simulink model "atrias_boom_nmSt_kinSw_v2"  (R2015a)
settings: Solver=ode23t  StartTime=0.0  StopTime=t_end  FixedStep=0.001  MaxStep=1e-3  RelTol=1e-3
InitFcn:
  | addpath('../common/')
  | colors
StartFcn:
  | tic
StopFcn:
  | %stopscript
values from neighbouring files (symbols this model uses):
  dt_a_dTrunk_boom = 5    [main_1_nmSt_kinSw.m]    (also in main_2_nmSt_kinSw_v2.m; main_3_nmSt_kinSw_v3.m; main_4_nmSt_kinSw_v4.m)
  dt_fade_boomCtrl = 2    [main_1_nmSt_kinSw.m]    (also in main_2_nmSt_kinSw_v2.m; main_3_nmSt_kinSw_v3.m; main_4_nmSt_kinSw_v4.m)
  initial_boom_yaw = 15*pi/180    (= 0.261799387799)    [main_2_nmSt_kinSw_v2.m]    (also in main_3_nmSt_kinSw_v3.m; main_4_nmSt_kinSw_v4.m)
  kd_boom_roll_Ctrl = 0    [main_1_nmSt_kinSw - Copy.m]    (also in main_1_nmSt_kinSw.m; main_2_nmSt_kinSw_v2.m; main_3_nmSt_kinSw_v3.m; main_4_nmSt_kinSw_v4.m)
  kd_boom_yaw_Ctrl = 0.1*kp_boom_yaw_Ctrl    (= 100000000)    [main_1_nmSt_kinSw - Copy.m]    (also in main_1_nmSt_kinSw.m = 1000000000; main_2_nmSt_kinSw_v2.m = 10000000; main_3_nmSt_kinSw_v3.m = 10000000; main_4_nmSt_kinSw_v4.m = 10000000)
  kd_motor = 0.90*2*sqrt(3.75*kp_motor)    [main_1_nmSt_kinSw - Copy.m]
  kinSw_alpha_start = 100*pi/180    (= 1.74532925199)    [main_1_nmSt_kinSw - Copy.m]    (also in main_1_nmSt_kinSw.m = 1.91986217719; main_2_nmSt_kinSw_v2.m = 1.83259571459; main_3_nmSt_kinSw_v3.m = 1.83259571459; main_4_nmSt_kinSw_v4.m = 1.83259571459)
  kinSw_alpha_tgt = 80*pi/180    (= 1.3962634016)    [main_1_nmSt_kinSw - Copy.m]    (also in main_1_nmSt_kinSw.m = 1.2217304764; main_2_nmSt_kinSw_v2.m = 1.2217304764; main_3_nmSt_kinSw_v3.m = 1.2217304764; main_4_nmSt_kinSw_v4.m = 1.2217304764)
  kinSw_t_start = 1.5    [main_1_nmSt_kinSw - Copy.m]    (also in main_1_nmSt_kinSw.m; main_2_nmSt_kinSw_v2.m = 0.5; main_3_nmSt_kinSw_v3.m = 0.5; main_4_nmSt_kinSw_v4.m = 0.5)
  kp_boom_roll_Ctrl = 0    [main_1_nmSt_kinSw - Copy.m]    (also in main_1_nmSt_kinSw.m; main_2_nmSt_kinSw_v2.m; main_3_nmSt_kinSw_v3.m; main_4_nmSt_kinSw_v4.m)
  kp_boom_yaw_Ctrl = 1e9    (= 1000000000)    [main_1_nmSt_kinSw - Copy.m]    (also in main_1_nmSt_kinSw.m = 10000000000; main_2_nmSt_kinSw_v2.m = 100000000; main_3_nmSt_kinSw_v3.m = 100000000; main_4_nmSt_kinSw_v4.m = 100000000)
  kp_motor = 3000    [main_1_nmSt_kinSw - Copy.m]
  max_back_bar_angle = 262.4*pi/180    (= 4.57974395723)    [main_1_nmSt_kinSw - Copy.m]
  max_front_bar_angle = 194.8*pi/180    (= 3.39990138288)    [main_1_nmSt_kinSw - Copy.m]
  min_back_bar_angle = 165.0*pi/180    (= 2.87979326579)    [main_1_nmSt_kinSw - Copy.m]
  min_front_bar_angle = 98.0*pi/180    (= 1.71042266695)    [main_1_nmSt_kinSw - Copy.m]
  poser_LLegAlp = (initial_l_leg_angle -pi/2)*180/pi    (= 105)    [main_2_nmSt_kinSw_v2.m]    (also in main_3_nmSt_kinSw_v3.m; main_4_nmSt_kinSw_v4.m)
  poser_LLegLen = initial_l_leg_length    (= 0.88)    [main_2_nmSt_kinSw_v2.m]    (also in main_3_nmSt_kinSw_v3.m; main_4_nmSt_kinSw_v4.m)
  poser_RLegAlp = (initial_r_leg_angle -pi/2)*180/pi    (= 75)    [main_2_nmSt_kinSw_v2.m]    (also in main_3_nmSt_kinSw_v3.m; main_4_nmSt_kinSw_v4.m)
  poser_RLegLen = initial_r_leg_length    (= 0.9)    [main_2_nmSt_kinSw_v2.m]    (also in main_3_nmSt_kinSw_v3.m; main_4_nmSt_kinSw_v4.m)
  tEnd_boomCtrl = t_end    (= 20)    [main_1_nmSt_kinSw - Copy.m]    (also in main_1_nmSt_kinSw.m = 3; main_2_nmSt_kinSw_v2.m = 7.5; main_3_nmSt_kinSw_v3.m = 7.5; main_4_nmSt_kinSw_v4.m = 7.5)
  tStart_boomCtrl = 1    [main_1_nmSt_kinSw - Copy.m]    (also in main_1_nmSt_kinSw.m = 0; main_2_nmSt_kinSw_v2.m = 0.5; main_3_nmSt_kinSw_v3.m = 0.5; main_4_nmSt_kinSw_v4.m = 0.5)
  tune_kinSw_alpha_start = kinSw_alpha_start*180/pi    (= 105)    [main_2_nmSt_kinSw_v2.m]    (also in main_3_nmSt_kinSw_v3.m; main_4_nmSt_kinSw_v4.m)
  tune_kinSw_alpha_tgt = kinSw_alpha_tgt*180/pi    (= 70)    [main_2_nmSt_kinSw_v2.m]    (also in main_3_nmSt_kinSw_v3.m; main_4_nmSt_kinSw_v4.m)
  tune_kinSw_len_min = kinSw_lclr    (= 0.7)    [main_2_nmSt_kinSw_v2.m]    (also in main_3_nmSt_kinSw_v3.m = 0.6)
  tune_kinSw_len_tgt = kinSw_len_tgt    (= 0.9)    [main_2_nmSt_kinSw_v2.m]    (also in main_3_nmSt_kinSw_v3.m)
  tune_M1_G = St_FGain_VAS*FmaxVAS    [main_2_nmSt_kinSw_v2.m]    (also in main_3_nmSt_kinSw_v3.m; main_4_nmSt_kinSw_v4.m)
  tune_M3_0 = CtrlPar_theta0*180/pi    [main_2_nmSt_kinSw_v2.m]    (also in main_3_nmSt_kinSw_v3.m; main_4_nmSt_kinSw_v4.m)
  tune_M3_D = St_GainDTh_HFL    [main_2_nmSt_kinSw_v2.m]    (also in main_3_nmSt_kinSw_v3.m; main_4_nmSt_kinSw_v4.m)
  tune_M3_P = St_GainTh_HFL    [main_2_nmSt_kinSw_v2.m]    (also in main_3_nmSt_kinSw_v3.m; main_4_nmSt_kinSw_v4.m)
  v_dTrunk_boom = 1.3    [main_1_nmSt_kinSw.m]    (also in main_2_nmSt_kinSw_v2.m; main_3_nmSt_kinSw_v3.m; main_4_nmSt_kinSw_v4.m)
undefined symbols (not defined in the file or in its folder): A1_notch_f1, A2_notch_f1, A_lpf_dtau, A_lpf_velocity, ankle_stiffness, B1_lpf_dtau, B1_lpf_velocity, B1_notch_f1, B2_lpf_dtau, B2_lpf_velocity, B2_notch_f1, b_hmotor, b_leg_spring, b_rotor, base_color_d, boom_color_d, boom_mount_to_center_diagonal, breakaway_friction, c_jointstop, contactThr, coulomb_friction, d_com, delta_phi_max, delta_phi_max_buffer, delta_phi_max_dropoff, delta_phi_min, fblink_color_d, floor_color_d, FmaxBFSH, FmaxGLU, FmaxHAM, FmaxHFL, FmaxRF, FmaxVAS, foot_color_d, FPCtrlPar, friction_linear_zone, g, gain_nodes_sea_torque, HIP_MTR_MAX_CONT_TORQUE, HIP_MTR_MAX_TORQUE, hshaft_color_d, initial_boom_pitch, initial_boom_roll, initial_hip_roll, initial_winch_angle, j_motor, k_gn, k_gt, k_leg_spring, K_notch_f1, k_phi, k_sea, Kb_leg, kd_lateral, kd_shin_max, kd_shin_min, kd_splay_max, kd_splay_min, kd_thigh_max ... (+187)
libraries: sm_lib x210, nesl_utility x140, simulink x65, simulink_extras x31, fl_lib x16, mblibv1 x2, commnoisgen2 x1
(part 3 of 16)

== system atrias_boom_nmSt_kinSw_v2/Mechanical System Layer/Left Foot ==
  Ankle : sm_lib/Joints/Revolute Joint  SenseConstraintForce=off  SenseConstraintForceX=off  SenseConstraintForceY=off  SenseConstraintForceZ=off  SenseConstraintTorque=off  SenseConstraintTorqueX=off  SenseConstraintTorqueY=off  SenseConstraintTorqueZ=off  SenseTotalForce=off  SenseTotalForceX=off  SenseTotalForceY=off  SenseTotalForceZ=off  SenseTotalTorque=off  SenseTotalTorqueX=off  SenseTotalTorqueY=off  SenseTotalTorqueZ=off  CompositeWrenchDir=FollowerOnBase  CompositeWrenchFrame=BaseFrame  EquilibriumPosition=ankle_equilibrium  EquilibriumPositionUnits=rad  SpringStiffness=ankle_stiffness  SpringStiffnessUnits=N*m/rad  DampingCoefficient=0.1*ankle_stiffness  DampingCoefficientUnits=N*m/(rad/s)  TorqueActuationMode=NoTorque  MotionActuationMode=ComputedMotion  SensePosition=off  SenseVelocity=off  SenseAcceleration=off  SenseTorqueForce=off  PositionTargetSpecify=on  PositionTargetPriority=Low  PositionTargetValue=ankle_initial_l  PositionTargetValueUnits=rad  VelocityTargetSpecify=off  VelocityTargetPriority=High  VelocityTargetValue=6000  VelocityTargetValueUnits=deg/s  BlockFunction=simmechanics.library.joints.revolute_joint
  CS1 to Back Point : sm_lib/Frames and Transforms/Rigid Transform  TranslationMethod=Cartesian  TranslationLengthUnit=m  TranslationStandardAxis=+Z  TranslationStandardOffset=0  TranslationCartesianOffset=d_foot_point_back  TranslationROffset=0  TranslationROffsetUnits=m  TranslationZOffset=0  TranslationZOffsetUnits=m  TranslationThetaOffset=0  TranslationThetaOffsetUnits=deg  RotationMethod=None  RotationAngleUnits=deg  RotationStandardAxis=+Z  RotationAngle=0  RotationArbitraryAxis=[0 0 1]  FollAlignAxisA=+X  BaseAlignAxisA=+Y  FollAlignAxisB=+Y  BaseAlignAxisB=+Z  RotationMatrix=[1 0 0; 0 1 0; 0 0 1]  BlockFunction=simmechanics.library.frames_transforms.rigid_transform
  CS1 to Front Point : sm_lib/Frames and Transforms/Rigid Transform  TranslationMethod=Cartesian  TranslationLengthUnit=m  TranslationStandardAxis=+Z  TranslationStandardOffset=0  TranslationCartesianOffset=d_foot_point_front  TranslationROffset=0  TranslationROffsetUnits=m  TranslationZOffset=0  TranslationZOffsetUnits=m  TranslationThetaOffset=0  TranslationThetaOffsetUnits=deg  RotationMethod=None  RotationAngleUnits=deg  RotationStandardAxis=+Z  RotationAngle=0  RotationArbitraryAxis=[0 0 1]  FollAlignAxisA=+X  BaseAlignAxisA=+Y  FollAlignAxisB=+Y  BaseAlignAxisB=+Z  RotationMatrix=[1 0 0; 0 1 0; 0 0 1]  BlockFunction=simmechanics.library.frames_transforms.rigid_transform
  Solid : sm_lib/Body Elements/Solid  InertiaType=Custom  Mass=m_foot  MassUnits=kg  CenterOfMass=com_foot  CenterOfMassUnits=m  MomentsOfInertia=i_foot_moments  MomentsOfInertiaUnits=kg*m^2  ProductsOfInertia=i_foot_products  ProductsOfInertiaUnits=kg*m^2  DensityBased=on  Density=1000  DensityUnits=kg/(m^3)  GraphicType=FromGeometry  MarkerShape=Sphere  MarkerSize=10  MarkerSizeUnits=m  GraphicVisPropType=AdvancedVisualProperties  GraphicDiffuseColor=foot_color_d  GraphicSpecularColor=[0.5 0.5 0.5 1.0]  GraphicAmbientColor=[foot_color_d*0.5 1.0]  GraphicEmissiveColor=[0.0 0.0 0.0 1.0]  GraphicShininess=128  GraphicOpacity=1.0  GeometryShape=FromFile  RectangleSize=[1 1]  RectangleSizeUnits=m  BrickDimensions=[0.1 l_seg 0.1]  BrickDimensionUnits=m  CylinderRadius=l_rad  CylinderRadiusUnits=m  CylinderLength=l_seg  CylinderLengthUnits=m  SphereRadius=1  SphereRadiusUnits=m  EllipsoidRadii=[1 1 1]  EllipsoidRadiiUnits=m  ExtrusionCrossSection=[1 1; -1 1; -1 -1; 1 -1]  ExtrusionCrossSectionUnits=m  ExtrusionLength=1  ExtrusionLengthUnits=m  PolygonNumSides=3  PolygonOuterRadius=1  PolygonOuterRadiusUnits=m  ExtGeomFileType=STL  ExtGeomFileName=../models/foot.stl  ExtGeomFileUnits=m  RevolutionCrossSection=[1 1; 1 -1; 2 -1; 2 1]  RevolutionCrossSectionUnits=m  RevolutionExtent=Full  RevolutionAngle=180  RevolutionAngleUnits=deg  BlockFunction=simmechanics.library.body_elements.solid
  CS1 : PMIOPort  Port=1  Side=Left
  Back Point : PMIOPort  Port=2  Side=Right
  Front Point : PMIOPort  Port=3  Side=Right
  connections:
  Front Point/RConn1 -- CS1 to Front Point/RConn1
  Ankle/LConn1 -- CS1/RConn1
  CS1 to Front Point/LConn1 -- Solid/RConn1 -- CS1 to Back Point/LConn1 -- Ankle/RConn1
  Back Point/RConn1 -- CS1 to Back Point/RConn1

== system atrias_boom_nmSt_kinSw_v2/Mechanical System Layer/Left Hip Roll Joint ==
  note: Hip Roll Mechanics
  Hip Motor [Nm] : Inport
  1 / Gear Ratio : Gain  Gain=1/N_h
  Common Gear : sm_lib/Gears and Couplings/Gears/Common Gear Constraint  GearType=External  SpecificationType=PitchCircleRadii  CenterDistance=20.0  CenterDistanceUnits=cm  GearRatio=1.0  BaseGearRadius=r_hip_gearhead  BaseGearRadiusUnits=m  FollGearRadius=r_hip_shaft  FollGearRadiusUnits=m  AssemblyGearRotation=Free  BlockFunction=simmechanics.library.gears_couplings_drives.gears.common_gear
  Constant : Constant  Value=pi
  Damping : Gain  Gain=b_hmotor
  Hip Motor Frame : sm_lib/Frames and Transforms/Rigid Transform  TranslationMethod=Cartesian  TranslationLengthUnit=m  TranslationStandardAxis=+Z  TranslationStandardOffset=0  TranslationCartesianOffset=[0 r_hip_gearhead+r_hip_shaft 0]  TranslationROffset=0  TranslationROffsetUnits=m  TranslationZOffset=0  TranslationZOffsetUnits=m  TranslationThetaOffset=0  TranslationThetaOffsetUnits=deg  RotationMethod=None  RotationAngleUnits=deg  RotationStandardAxis=-Z  RotationAngle=180  RotationArbitraryAxis=[0 0 1]  FollAlignAxisA=+X  BaseAlignAxisA=+Z  FollAlignAxisB=+Y  BaseAlignAxisB=+Y  RotationMatrix=[1 0 0; 0 1 0; 0 0 1]  BlockFunction=simmechanics.library.frames_transforms.rigid_transform
  Hip Roll Frame : sm_lib/Frames and Transforms/Rigid Transform  TranslationMethod=None  TranslationLengthUnit=m  TranslationStandardAxis=+Z  TranslationStandardOffset=0  TranslationCartesianOffset=[0 0 0]  TranslationROffset=0  TranslationROffsetUnits=m  TranslationZOffset=0  TranslationZOffsetUnits=m  TranslationThetaOffset=0  TranslationThetaOffsetUnits=deg  RotationMethod=AlignedAxes  RotationAngleUnits=deg  RotationStandardAxis=-Z  RotationAngle=180  RotationArbitraryAxis=[0 0 1]  FollAlignAxisA=-X  BaseAlignAxisA=+Z  FollAlignAxisB=+Y  BaseAlignAxisB=+Y  RotationMatrix=[1 0 0; 0 1 0; 0 0 1]  BlockFunction=simmechanics.library.frames_transforms.rigid_transform
  Hip Roll Joint : sm_lib/Joints/Revolute Joint  SenseConstraintForce=off  SenseConstraintForceX=off  SenseConstraintForceY=off  SenseConstraintForceZ=off  SenseConstraintTorque=off  SenseConstraintTorqueX=off  SenseConstraintTorqueY=off  SenseConstraintTorqueZ=off  SenseTotalForce=off  SenseTotalForceX=off  SenseTotalForceY=off  SenseTotalForceZ=off  SenseTotalTorque=off  SenseTotalTorqueX=off  SenseTotalTorqueY=off  SenseTotalTorqueZ=off  CompositeWrenchDir=FollowerOnBase  CompositeWrenchFrame=BaseFrame  EquilibriumPosition=0  EquilibriumPositionUnits=deg  SpringStiffness=0  SpringStiffnessUnits=N*m/deg  DampingCoefficient=0  DampingCoefficientUnits=N*m/(deg/s)  TorqueActuationMode=InputTorque  MotionActuationMode=ComputedMotion  SensePosition=on  SenseVelocity=on  SenseAcceleration=off  SenseTorqueForce=off  PositionTargetSpecify=on  PositionTargetPriority=High  PositionTargetValue=initial_hip_roll  PositionTargetValueUnits=rad  VelocityTargetSpecify=off  VelocityTargetPriority=High  VelocityTargetValue=0  VelocityTargetValueUnits=deg/s  BlockFunction=simmechanics.library.joints.revolute_joint
  Leg Frame : sm_lib/Frames and Transforms/Rigid Transform  TranslationMethod=None  TranslationLengthUnit=m  TranslationStandardAxis=+Z  TranslationStandardOffset=0  TranslationCartesianOffset=[0 0 0]  TranslationROffset=0  TranslationROffsetUnits=m  TranslationZOffset=0  TranslationZOffsetUnits=m  TranslationThetaOffset=0  TranslationThetaOffsetUnits=deg  RotationMethod=AlignedAxes  RotationAngleUnits=deg  RotationStandardAxis=-Z  RotationAngle=180  RotationArbitraryAxis=[0 0 1]  FollAlignAxisA=+Z  BaseAlignAxisA=-X  FollAlignAxisB=+Y  BaseAlignAxisB=+Y  RotationMatrix=[1 0 0; 0 1 0; 0 0 1]  BlockFunction=simmechanics.library.frames_transforms.rigid_transform
  "Mechanical Limits " : Subsystem
  Motor Efficiency : Gain  Gain=mu_hmotor
  Motor Joint : sm_lib/Joints/Revolute Joint  SenseConstraintForce=off  SenseConstraintForceX=off  SenseConstraintForceY=off  SenseConstraintForceZ=off  SenseConstraintTorque=off  SenseConstraintTorqueX=off  SenseConstraintTorqueY=off  SenseConstraintTorqueZ=off  SenseTotalForce=off  SenseTotalForceX=off  SenseTotalForceY=off  SenseTotalForceZ=off  SenseTotalTorque=off  SenseTotalTorqueX=off  SenseTotalTorqueY=off  SenseTotalTorqueZ=off  CompositeWrenchDir=FollowerOnBase  CompositeWrenchFrame=BaseFrame  EquilibriumPosition=0  EquilibriumPositionUnits=deg  SpringStiffness=0  SpringStiffnessUnits=N*m/deg  DampingCoefficient=0  DampingCoefficientUnits=N*m/(deg/s)  TorqueActuationMode=InputTorque  MotionActuationMode=ComputedMotion  SensePosition=off  SenseVelocity=on  SenseAcceleration=off  SenseTorqueForce=off  PositionTargetSpecify=off  PositionTargetPriority=Low  PositionTargetValue=30  PositionTargetValueUnits=deg  VelocityTargetSpecify=off  VelocityTargetPriority=High  VelocityTargetValue=0  VelocityTargetValueUnits=deg/s  BlockFunction=simmechanics.library.joints.revolute_joint
  PS-Simulink Converter : nesl_utility/PS-Simulink Converter  PhysicalDomain=network_engine_domain  SubClassName=ps_output  LeftPortType=input  RightPortType=output  PseudoPeriodic=off  Frequencies=[]  Unit=1  AffineConversion=off
  PS-Simulink Converter1 : nesl_utility/PS-Simulink Converter  PhysicalDomain=network_engine_domain  SubClassName=ps_output  LeftPortType=input  RightPortType=output  PseudoPeriodic=off  Frequencies=[]  Unit=1  AffineConversion=off
  PS-Simulink Converter3 : nesl_utility/PS-Simulink Converter  PhysicalDomain=network_engine_domain  SubClassName=ps_output  LeftPortType=input  RightPortType=output  PseudoPeriodic=off  Frequencies=[]  Unit=1  AffineConversion=off
  Rotor : sm_lib/Body Elements/Solid  InertiaType=Custom  Mass=0  MassUnits=kg  CenterOfMass=[0 0 0]  CenterOfMassUnits=m  MomentsOfInertia=i_hrotor_moments  MomentsOfInertiaUnits=kg*m^2  ProductsOfInertia=[0 0 0]  ProductsOfInertiaUnits=kg*m^2  DensityBased=on  Density=1000  DensityUnits=kg/(m^3)  GraphicType=None  MarkerShape=Sphere  MarkerSize=10  MarkerSizeUnits=m  GraphicVisPropType=AdvancedVisualProperties  GraphicDiffuseColor=hshaft_color_d  GraphicSpecularColor=[0.5 0.5 0.5 1.0]  GraphicAmbientColor=[0.15 0.15 0.15 1.0]  GraphicEmissiveColor=[0.0 0.0 0.0 1.0]  GraphicShininess=10  GraphicOpacity=1.0  GeometryShape=Cylinder  RectangleSize=[1 1]  RectangleSizeUnits=m  BrickDimensions=[1 1 1]  BrickDimensionUnits=m  CylinderRadius=0.1  CylinderRadiusUnits=m  CylinderLength=0.1  CylinderLengthUnits=m  SphereRadius=1  SphereRadiusUnits=m  EllipsoidRadii=[1 1 1]  EllipsoidRadiiUnits=m  ExtrusionCrossSection=[1 1; -1 1; -1 -1; 1 -1]  ExtrusionCrossSectionUnits=m  ExtrusionLength=1  ExtrusionLengthUnits=m  PolygonNumSides=3  PolygonOuterRadius=1  PolygonOuterRadiusUnits=m  ExtGeomFileType=STL  ExtGeomFileUnits=m  RevolutionCrossSection=[1 1; 1 -1; 2 -1; 2 1]  RevolutionCrossSectionUnits=m  RevolutionExtent=Full  RevolutionAngle=180  RevolutionAngleUnits=deg  BlockFunction=simmechanics.library.body_elements.solid
  Simulink-PS Converter : nesl_utility/Simulink-PS Converter  PhysicalDomain=network_engine_domain  SubClassName=ps_input  LeftPortType=input  RightPortType=output  PseudoPeriodic=off  Frequencies=[]  NoiseDistribution=none  NoiseParameters=[]  Unit=1  AffineConversion=off  InputFiltering=off  SimscapeFilterOrder=1  InputFilterTimeConstant=0.001  UdotUserProvided=1
  Simulink-PS Converter1 : nesl_utility/Simulink-PS Converter  PhysicalDomain=network_engine_domain  SubClassName=ps_input  LeftPortType=input  RightPortType=output  PseudoPeriodic=off  Frequencies=[]  NoiseDistribution=none  NoiseParameters=[]  Unit=1  AffineConversion=off  InputFiltering=off  SimscapeFilterOrder=1  InputFilterTimeConstant=0.001  UdotUserProvided=1
  Sum : Sum  Inputs=|+-
  Sum1 : Sum  Inputs=++|
  Torque Limiter (outside) 1 : Saturate  UpperLimit=HIP_MTR_MAX_TORQUE  LowerLimit=-HIP_MTR_MAX_TORQUE  ZeroCross=off
      settings: AttributesFormatString=Hi: %<UpperLimit>\nLo: %<LowerLimit>
  Leg Hip Conn : PMIOPort  Port=1  Side=Left
  Torso Hip Conn : PMIOPort  Port=2  Side=Right
  Hip Roll [rad] : Outport
  wires:
  Sum1/1 -> "Mechanical Limits "/2(phi)
  PS-Simulink Converter1/1 -> "Mechanical Limits "/1(vphi)
  "Mechanical Limits "/1(tau_reaction) -> Simulink-PS Converter/1
  1 / Gear Ratio/1 -> Sum/1
  Hip Motor [Nm]/1 -> Torque Limiter (outside) 1/1
  Constant/1 -> Sum1/2
  PS-Simulink Converter3/1 -> Damping/1
  Damping/1 -> Sum/2
  Sum/1 -> Motor Efficiency/1
  PS-Simulink Converter/1 -> Hip Roll [rad]/1, Sum1/1
  Motor Efficiency/1 -> Simulink-PS Converter1/1
  Torque Limiter (outside) 1/1 -> 1 / Gear Ratio/1
  connections:
  Motor Joint/RConn1 -- Common Gear/LConn1 -- Rotor/RConn1
  Hip Motor Frame/RConn1 -- Motor Joint/LConn1
  Hip Roll Joint/RConn1 -- Common Gear/RConn1 -- Leg Frame/LConn1
  Simulink-PS Converter1/RConn1 -- Motor Joint/LConn2
  Motor Joint/RConn2 -- PS-Simulink Converter3/LConn1
  Leg Frame/RConn1 -- Leg Hip Conn/RConn1
  Hip Roll Frame/LConn1 -- Torso Hip Conn/RConn1
  PS-Simulink Converter1/LConn1 -- Hip Roll Joint/RConn3
  PS-Simulink Converter/LConn1 -- Hip Roll Joint/RConn2
  Simulink-PS Converter/RConn1 -- Hip Roll Joint/LConn2
  Hip Roll Joint/LConn1 -- Hip Roll Frame/RConn1 -- Hip Motor Frame/LConn1

== system atrias_boom_nmSt_kinSw_v2/Mechanical System Layer/Pitch Joint ==
  PS-Simulink Converter3 : nesl_utility/PS-Simulink Converter  PhysicalDomain=network_engine_domain  SubClassName=ps_output  LeftPortType=input  RightPortType=output  PseudoPeriodic=off  Frequencies=[]  Unit=1  AffineConversion=off
  Pitch Joint : sm_lib/Joints/Revolute Joint  SenseConstraintForce=off  SenseConstraintForceX=off  SenseConstraintForceY=off  SenseConstraintForceZ=off  SenseConstraintTorque=off  SenseConstraintTorqueX=off  SenseConstraintTorqueY=off  SenseConstraintTorqueZ=off  SenseTotalForce=off  SenseTotalForceX=off  SenseTotalForceY=off  SenseTotalForceZ=off  SenseTotalTorque=off  SenseTotalTorqueX=off  SenseTotalTorqueY=off  SenseTotalTorqueZ=off  CompositeWrenchDir=FollowerOnBase  CompositeWrenchFrame=BaseFrame  EquilibriumPosition=0  EquilibriumPositionUnits=deg  SpringStiffness=0  SpringStiffnessUnits=N*m/rad  DampingCoefficient=0  DampingCoefficientUnits=N*m/(rad/s)  TorqueActuationMode=NoTorque  MotionActuationMode=ComputedMotion  SensePosition=on  SenseVelocity=off  SenseAcceleration=off  SenseTorqueForce=off  PositionTargetSpecify=on  PositionTargetPriority=High  PositionTargetValue=initial_boom_pitch  PositionTargetValueUnits=rad  VelocityTargetSpecify=off  VelocityTargetPriority=High  VelocityTargetValue=0  VelocityTargetValueUnits=deg/s  BlockFunction=simmechanics.library.joints.revolute_joint
  Pitch Mount Slant : sm_lib/Frames and Transforms/Rigid Transform  TranslationMethod=None  TranslationLengthUnit=m  TranslationStandardAxis=+Z  TranslationStandardOffset=0  TranslationCartesianOffset=[0 0 0]  TranslationROffset=0  TranslationROffsetUnits=m  TranslationZOffset=0  TranslationZOffsetUnits=m  TranslationThetaOffset=0  TranslationThetaOffsetUnits=deg  RotationMethod=ArbitraryAxis  RotationAngleUnits=rad  RotationStandardAxis=+Z  RotationAngle=pitch_mount_angle  RotationArbitraryAxis=[-1 0 0]  FollAlignAxisA=+X  BaseAlignAxisA=+Y  FollAlignAxisB=+Y  BaseAlignAxisB=+Z  RotationMatrix=[1 0 0; 0 1 0; 0 0 1]  BlockFunction=simmechanics.library.frames_transforms.rigid_transform
  Pitch Orientation : sm_lib/Frames and Transforms/Rigid Transform  TranslationMethod=None  TranslationLengthUnit=m  TranslationStandardAxis=+Z  TranslationStandardOffset=0  TranslationCartesianOffset=[0 0 0]  TranslationROffset=0  TranslationROffsetUnits=m  TranslationZOffset=0  TranslationZOffsetUnits=m  TranslationThetaOffset=0  TranslationThetaOffsetUnits=deg  RotationMethod=AlignedAxes  RotationAngleUnits=rad  RotationStandardAxis=+Z  RotationAngle=0  RotationArbitraryAxis=[-1 0 0]  FollAlignAxisA=+Z  BaseAlignAxisA=-Z  FollAlignAxisB=+Y  BaseAlignAxisB=+Y  RotationMatrix=[1 0 0; 0 1 0; 0 0 1]  BlockFunction=simmechanics.library.frames_transforms.rigid_transform
  World Orientation : sm_lib/Frames and Transforms/Rigid Transform  TranslationMethod=None  TranslationLengthUnit=m  TranslationStandardAxis=+Z  TranslationStandardOffset=0  TranslationCartesianOffset=[0 0 0]  TranslationROffset=0  TranslationROffsetUnits=m  TranslationZOffset=0  TranslationZOffsetUnits=m  TranslationThetaOffset=0  TranslationThetaOffsetUnits=deg  RotationMethod=AlignedAxes  RotationAngleUnits=rad  RotationStandardAxis=+Z  RotationAngle=0  RotationArbitraryAxis=[-1 0 0]  FollAlignAxisA=+Z  BaseAlignAxisA=-Z  FollAlignAxisB=+Y  BaseAlignAxisB=+Y  RotationMatrix=[1 0 0; 0 1 0; 0 0 1]  BlockFunction=simmechanics.library.frames_transforms.rigid_transform
  Boom : PMIOPort  Port=1  Side=Right
  Torso : PMIOPort  Port=2  Side=Left
  Pitch [rad] : Outport
  wires:
  PS-Simulink Converter3/1 -> Pitch [rad]/1
  connections:
  Pitch Orientation/RConn1 -- Pitch Joint/LConn1
  PS-Simulink Converter3/LConn1 -- Pitch Joint/RConn2
  Boom/RConn1 -- Pitch Mount Slant/LConn1
  World Orientation/RConn1 -- Torso/RConn1
  Pitch Orientation/LConn1 -- Pitch Mount Slant/RConn1
  Pitch Joint/RConn1 -- World Orientation/LConn1

== system atrias_boom_nmSt_kinSw_v2/Mechanical System Layer/R Hip Shaft ==
  CS1 to CS2 : sm_lib/Frames and Transforms/Rigid Transform  TranslationMethod=Cartesian  TranslationLengthUnit=m  TranslationStandardAxis=+Z  TranslationStandardOffset=0  TranslationCartesianOffset=hshaft_12  TranslationROffset=0  TranslationROffsetUnits=m  TranslationZOffset=0  TranslationZOffsetUnits=m  TranslationThetaOffset=0  TranslationThetaOffsetUnits=deg  RotationMethod=None  RotationAngleUnits=deg  RotationStandardAxis=+Z  RotationAngle=0  RotationArbitraryAxis=[0 0 1]  FollAlignAxisA=+X  BaseAlignAxisA=+Y  FollAlignAxisB=+Y  BaseAlignAxisB=+Z  RotationMatrix=[1 0 0; 0 1 0; 0 0 1]  BlockFunction=simmechanics.library.frames_transforms.rigid_transform
  Frame Data : Subsystem
  Solid : sm_lib/Body Elements/Solid  InertiaType=Custom  Mass=m_hshaft  MassUnits=kg  CenterOfMass=com_hshaft  CenterOfMassUnits=m  MomentsOfInertia=i_hshaft_moments  MomentsOfInertiaUnits=kg*m^2  ProductsOfInertia=i_hshaft_products  ProductsOfInertiaUnits=kg*m^2  DensityBased=on  Density=1000  DensityUnits=kg/(m^3)  GraphicType=FromGeometry  MarkerShape=Sphere  MarkerSize=10  MarkerSizeUnits=m  GraphicVisPropType=AdvancedVisualProperties  GraphicDiffuseColor=hshaft_color_d  GraphicSpecularColor=[[1 1 1]*0.5 1.0]  GraphicAmbientColor=[hshaft_color_d*0.50 1.0]  GraphicEmissiveColor=[0 0 0 1.0]  GraphicShininess=128  GraphicOpacity=1.0  GeometryShape=FromFile  RectangleSize=[1 1]  RectangleSizeUnits=m  BrickDimensions=[1 1 1]  BrickDimensionUnits=m  CylinderRadius=l_rad  CylinderRadiusUnits=m  CylinderLength=l_seg  CylinderLengthUnits=m  SphereRadius=1  SphereRadiusUnits=m  EllipsoidRadii=[1 1 1]  EllipsoidRadiiUnits=m  ExtrusionCrossSection=[1 1; -1 1; -1 -1; 1 -1]  ExtrusionCrossSectionUnits=m  ExtrusionLength=1  ExtrusionLengthUnits=m  PolygonNumSides=3  PolygonOuterRadius=1  PolygonOuterRadiusUnits=m  ExtGeomFileType=STL  ExtGeomFileName=../models/hip_shaft.STL  ExtGeomFileUnits=m  RevolutionCrossSection=[1 1; 1 -1; 2 -1; 2 1]  RevolutionCrossSectionUnits=m  RevolutionExtent=Full  RevolutionAngle=180  RevolutionAngleUnits=deg  BlockFunction=simmechanics.library.body_elements.solid
  CS1 : PMIOPort  Port=1  Side=Right
  CS2 : PMIOPort  Port=2  Side=Left
  connections:
  CS1/RConn1 -- Frame Data/LConn1 -- Solid/RConn1 -- CS1 to CS2/LConn1
  CS2/RConn1 -- CS1 to CS2/RConn1

== system atrias_boom_nmSt_kinSw_v2/Mechanical System Layer/R Leg ==
  Shin Motor [Nm] : Inport
  "Thigh Motor [Nm]  " : Inport  Port=2
  Angle Range Map : Subsystem
  Angle Range Map1 : Subsystem
  Anterior Knee : sm_lib/Joints/Revolute Joint  SenseConstraintForce=off  SenseConstraintForceX=off  SenseConstraintForceY=off  SenseConstraintForceZ=off  SenseConstraintTorque=off  SenseConstraintTorqueX=off  SenseConstraintTorqueY=off  SenseConstraintTorqueZ=off  SenseTotalForce=off  SenseTotalForceX=off  SenseTotalForceY=off  SenseTotalForceZ=off  SenseTotalTorque=off  SenseTotalTorqueX=off  SenseTotalTorqueY=off  SenseTotalTorqueZ=off  CompositeWrenchDir=FollowerOnBase  CompositeWrenchFrame=BaseFrame  EquilibriumPosition=0  EquilibriumPositionUnits=deg  SpringStiffness=0  SpringStiffnessUnits=N*m/deg  DampingCoefficient=0  DampingCoefficientUnits=N*m/(deg/s)  TorqueActuationMode=NoTorque  MotionActuationMode=ComputedMotion  SensePosition=off  SenseVelocity=off  SenseAcceleration=off  SenseTorqueForce=off  PositionTargetSpecify=off  PositionTargetPriority=Low  PositionTargetValue=30  PositionTargetValueUnits=deg  VelocityTargetSpecify=off  VelocityTargetPriority=High  VelocityTargetValue=0  VelocityTargetValueUnits=deg/s  BlockFunction=simmechanics.library.joints.revolute_joint
  External Force and Torque1 : sm_lib/Forces and Torques/External Force and Torque  ForceResolutionFrame=AttachedFrame  EnableForceX=off  EnableForceY=off  EnableForceZ=off  EnableForce=off  TorqueResolutionFrame=AttachedFrame  EnableTorqueX=off  EnableTorqueY=off  EnableTorqueZ=on  EnableTorque=off  BlockFunction=simmechanics.library.forces_torques.external_force_torque
  External Force and Torque2 : sm_lib/Forces and Torques/External Force and Torque  ForceResolutionFrame=AttachedFrame  EnableForceX=off  EnableForceY=off  EnableForceZ=off  EnableForce=off  TorqueResolutionFrame=AttachedFrame  EnableTorqueX=off  EnableTorqueY=off  EnableTorqueZ=on  EnableTorque=off  BlockFunction=simmechanics.library.forces_torques.external_force_torque
  Flip Rotation Direction : sm_lib/Frames and Transforms/Rigid Transform  TranslationMethod=None  TranslationLengthUnit=m  TranslationStandardAxis=+Z  TranslationStandardOffset=0  TranslationCartesianOffset=[0 0 0]  TranslationROffset=0  TranslationROffsetUnits=m  TranslationZOffset=0  TranslationZOffsetUnits=m  TranslationThetaOffset=0  TranslationThetaOffsetUnits=deg  RotationMethod=AlignedAxes  RotationAngleUnits=deg  RotationStandardAxis=-Z  RotationAngle=180  RotationArbitraryAxis=[0 0 1]  FollAlignAxisA=-Z  BaseAlignAxisA=+Z  FollAlignAxisB=+Y  BaseAlignAxisB=+Y  RotationMatrix=[1 0 0; 0 1 0; 0 0 1]  BlockFunction=simmechanics.library.frames_transforms.rigid_transform
  Flip Rotation Direction 1 : sm_lib/Frames and Transforms/Rigid Transform  TranslationMethod=None  TranslationLengthUnit=m  TranslationStandardAxis=+Z  TranslationStandardOffset=0  TranslationCartesianOffset=[0 0 0]  TranslationROffset=0  TranslationROffsetUnits=m  TranslationZOffset=0  TranslationZOffsetUnits=m  TranslationThetaOffset=0  TranslationThetaOffsetUnits=deg  RotationMethod=AlignedAxes  RotationAngleUnits=deg  RotationStandardAxis=-Z  RotationAngle=180  RotationArbitraryAxis=[0 0 1]  FollAlignAxisA=-Z  BaseAlignAxisA=+Z  FollAlignAxisB=+Y  BaseAlignAxisB=+Y  RotationMatrix=[1 0 0; 0 1 0; 0 0 1]  BlockFunction=simmechanics.library.frames_transforms.rigid_transform
  Flip Rotation Direction 2 : sm_lib/Frames and Transforms/Rigid Transform  TranslationMethod=None  TranslationLengthUnit=m  TranslationStandardAxis=+Z  TranslationStandardOffset=0  TranslationCartesianOffset=[0 0 0]  TranslationROffset=0  TranslationROffsetUnits=m  TranslationZOffset=0  TranslationZOffsetUnits=m  TranslationThetaOffset=0  TranslationThetaOffsetUnits=deg  RotationMethod=AlignedAxes  RotationAngleUnits=deg  RotationStandardAxis=-Z  RotationAngle=180  RotationArbitraryAxis=[0 0 1]  FollAlignAxisA=-Z  BaseAlignAxisA=+Z  FollAlignAxisB=+Y  BaseAlignAxisB=+Y  RotationMatrix=[1 0 0; 0 1 0; 0 0 1]  BlockFunction=simmechanics.library.frames_transforms.rigid_transform
  Four Bar Link : Subsystem
      mask Display: image('../images/fourbarlink.JPG');
  Four Bar Link Joint : sm_lib/Joints/Revolute Joint  SenseConstraintForce=off  SenseConstraintForceX=off  SenseConstraintForceY=off  SenseConstraintForceZ=off  SenseConstraintTorque=off  SenseConstraintTorqueX=off  SenseConstraintTorqueY=off  SenseConstraintTorqueZ=off  SenseTotalForce=off  SenseTotalForceX=off  SenseTotalForceY=off  SenseTotalForceZ=off  SenseTotalTorque=off  SenseTotalTorqueX=off  SenseTotalTorqueY=off  SenseTotalTorqueZ=off  CompositeWrenchDir=FollowerOnBase  CompositeWrenchFrame=BaseFrame  EquilibriumPosition=0  EquilibriumPositionUnits=deg  SpringStiffness=0  SpringStiffnessUnits=N*m/deg  DampingCoefficient=0  DampingCoefficientUnits=N*m/(deg/s)  TorqueActuationMode=NoTorque  MotionActuationMode=ComputedMotion  SensePosition=off  SenseVelocity=off  SenseAcceleration=off  SenseTorqueForce=off  PositionTargetSpecify=off  PositionTargetPriority=Low  PositionTargetValue=30  PositionTargetValueUnits=deg  VelocityTargetSpecify=off  VelocityTargetPriority=High  VelocityTargetValue=0  VelocityTargetValueUnits=deg/s  BlockFunction=simmechanics.library.joints.revolute_joint
  Gain : Gain  Gain=-1
  Lower Leg : Subsystem
      mask Display: image('../images/lowerleg.JPG');
  Mechanical Limits : Subsystem
      settings: MinAlgLoopOccurrences=on
  Mux1 : Mux  Inputs=2
  Mux2 : Mux  Inputs=2
  PS-Simulink Converter{,1..3} (4 alike) : nesl_utility/PS-Simulink Converter  PhysicalDomain=network_engine_domain  SubClassName=ps_output  LeftPortType=input  RightPortType=output  PseudoPeriodic=off  Frequencies=[]  Unit=1  AffineConversion=off
  Posterior Knee : sm_lib/Joints/Revolute Joint  SenseConstraintForce=off  SenseConstraintForceX=off  SenseConstraintForceY=off  SenseConstraintForceZ=off  SenseConstraintTorque=off  SenseConstraintTorqueX=off  SenseConstraintTorqueY=off  SenseConstraintTorqueZ=off  SenseTotalForce=off  SenseTotalForceX=off  SenseTotalForceY=off  SenseTotalForceZ=off  SenseTotalTorque=off  SenseTotalTorqueX=off  SenseTotalTorqueY=off  SenseTotalTorqueZ=off  CompositeWrenchDir=FollowerOnBase  CompositeWrenchFrame=BaseFrame  EquilibriumPosition=0  EquilibriumPositionUnits=deg  SpringStiffness=0  SpringStiffnessUnits=N*m/deg  DampingCoefficient=0  DampingCoefficientUnits=N*m/(deg/s)  TorqueActuationMode=NoTorque  MotionActuationMode=ComputedMotion  SensePosition=off  SenseVelocity=off  SenseAcceleration=off  SenseTorqueForce=off  PositionTargetSpecify=off  PositionTargetPriority=Low  PositionTargetValue=30  PositionTargetValueUnits=deg  VelocityTargetSpecify=off  VelocityTargetPriority=High  VelocityTargetValue=0  VelocityTargetValueUnits=deg/s  BlockFunction=simmechanics.library.joints.revolute_joint
  Rotate Frame 180 degrees : sm_lib/Frames and Transforms/Rigid Transform  TranslationMethod=None  TranslationLengthUnit=m  TranslationStandardAxis=+Z  TranslationStandardOffset=0  TranslationCartesianOffset=[0 0 0]  TranslationROffset=0  TranslationROffsetUnits=m  TranslationZOffset=0  TranslationZOffsetUnits=m  TranslationThetaOffset=0  TranslationThetaOffsetUnits=deg  RotationMethod=StandardAxis  RotationAngleUnits=deg  RotationStandardAxis=+Z  RotationAngle=180  RotationArbitraryAxis=[0 0 1]  FollAlignAxisA=-Z  BaseAlignAxisA=+Z  FollAlignAxisB=+Y  BaseAlignAxisB=+Y  RotationMatrix=[1 0 0; 0 1 0; 0 0 1]  BlockFunction=simmechanics.library.frames_transforms.rigid_transform
  Shin : Subsystem
      mask Display: image('../images/shin.JPG');
  Shin Joint : sm_lib/Joints/Revolute Joint  SenseConstraintForce=off  SenseConstraintForceX=off  SenseConstraintForceY=off  SenseConstraintForceZ=off  SenseConstraintTorque=off  SenseConstraintTorqueX=off  SenseConstraintTorqueY=off  SenseConstraintTorqueZ=off  SenseTotalForce=off  SenseTotalForceX=off  SenseTotalForceY=off  SenseTotalForceZ=off  SenseTotalTorque=off  SenseTotalTorqueX=off  SenseTotalTorqueY=off  SenseTotalTorqueZ=off  CompositeWrenchDir=FollowerOnBase  CompositeWrenchFrame=BaseFrame  EquilibriumPosition=0  EquilibriumPositionUnits=deg  SpringStiffness=0  SpringStiffnessUnits=N*m/deg  DampingCoefficient=0  DampingCoefficientUnits=N*m/(deg/s)  TorqueActuationMode=NoTorque  MotionActuationMode=ComputedMotion  SensePosition=on  SenseVelocity=on  SenseAcceleration=off  SenseTorqueForce=off  PositionTargetSpecify=on  PositionTargetPriority=High  PositionTargetValue=shin_initial_r  PositionTargetValueUnits=rad  VelocityTargetSpecify=on  VelocityTargetPriority=High  VelocityTargetValue=v_shin_initial_r  VelocityTargetValueUnits=rad/s  BlockFunction=simmechanics.library.joints.revolute_joint
  Shin SEA : Subsystem
      mask Display: image('../images/shinsea.JPG')
  Simulink-PS Converter : nesl_utility/Simulink-PS Converter  PhysicalDomain=network_engine_domain  SubClassName=ps_input  LeftPortType=input  RightPortType=output  PseudoPeriodic=off  Frequencies=[]  NoiseDistribution=none  NoiseParameters=[]  Unit=1  AffineConversion=off  InputFiltering=off  SimscapeFilterOrder=1  InputFilterTimeConstant=0.001  UdotUserProvided=1
  Simulink-PS Converter1 : nesl_utility/Simulink-PS Converter  PhysicalDomain=network_engine_domain  SubClassName=ps_input  LeftPortType=input  RightPortType=output  PseudoPeriodic=off  Frequencies=[]  NoiseDistribution=none  NoiseParameters=[]  Unit=1  AffineConversion=off  InputFiltering=off  SimscapeFilterOrder=1  InputFilterTimeConstant=0.001  UdotUserProvided=1
  Sum : Sum  Inputs=+|+
  Sum1 : Sum  Inputs=+|+
  Sum3 : Sum  Inputs=++|
  Sum4 : Sum  Inputs=++|
  Thigh : Subsystem
      mask Display: image('../images/thigh.JPG');
  Thigh Joint : sm_lib/Joints/Revolute Joint  SenseConstraintForce=off  SenseConstraintForceX=off  SenseConstraintForceY=off  SenseConstraintForceZ=off  SenseConstraintTorque=off  SenseConstraintTorqueX=off  SenseConstraintTorqueY=off  SenseConstraintTorqueZ=off  SenseTotalForce=off  SenseTotalForceX=off  SenseTotalForceY=off  SenseTotalForceZ=off  SenseTotalTorque=off  SenseTotalTorqueX=off  SenseTotalTorqueY=off  SenseTotalTorqueZ=off  CompositeWrenchDir=FollowerOnBase  CompositeWrenchFrame=BaseFrame  EquilibriumPosition=0  EquilibriumPositionUnits=deg  SpringStiffness=0  SpringStiffnessUnits=N*m/deg  DampingCoefficient=0  DampingCoefficientUnits=N*m/(deg/s)  TorqueActuationMode=NoTorque  MotionActuationMode=ComputedMotion  SensePosition=on  SenseVelocity=on  SenseAcceleration=off  SenseTorqueForce=off  PositionTargetSpecify=on  PositionTargetPriority=High  PositionTargetValue=thigh_initial_r  PositionTargetValueUnits=rad  VelocityTargetSpecify=on  VelocityTargetPriority=High  VelocityTargetValue=v_thigh_initial_r  VelocityTargetValueUnits=rad/s  BlockFunction=simmechanics.library.joints.revolute_joint
  Thigh SEA : Subsystem
      mask Display: image('../images/thighsea.JPG')
  Hip Conn : PMIOPort  Port=1  Side=Right
  Foot Point : PMIOPort  Port=2  Side=Left
  Shin Joint [rad] : Outport
  Shin Gear [rad] : Outport  Port=2
  Thigh Joint [rad] : Outport  Port=3
  Thigh Gear [rad] : Outport  Port=4
  wires:
  Angle Range Map1/1("[0,2*pi]") -> Mux1/1, Thigh Joint [rad]/1, Mechanical Limits/4(phi_thigh)
  Mux2/1 -> Shin SEA/2(Shin Joint [rad rad/s])
  Sum/1 -> Simulink-PS Converter/1
  Sum4/1 -> Sum/2
  Sum3/1 -> Sum1/1
  Mechanical Limits/1(tau_shin_col) -> Sum4/1
  Mechanical Limits/3(tau_thigh_col) -> Sum3/1
  Gain/1 -> Sum3/2
  Shin SEA/2(Shin Gear [rad]) -> Shin Gear [rad]/1
  Thigh SEA/2(Thigh Gear [rad]) -> Thigh Gear [rad]/1
  Mux1/1 -> Thigh SEA/2(Thigh Joint [rad rad/s])
  PS-Simulink Converter1/1 -> Mux2/2, Mechanical Limits/1(dphi_shin)
  Mechanical Limits/2(tau_thigh_shin_col) -> Sum4/2, Gain/1
  PS-Simulink Converter3/1 -> Mux1/2, Mechanical Limits/3(dphi_thigh)
  Thigh SEA/1(Thigh Joint Torque [Nm]) -> Sum1/2
  Sum1/1 -> Simulink-PS Converter1/1
  Shin SEA/1(Shin Joint Torque [Nm]) -> Sum/1
  PS-Simulink Converter2/1 -> Angle Range Map1/1("[-pi, pi]")
  Angle Range Map/1("[0,2*pi]") -> Mux2/1, Shin Joint [rad]/1, Mechanical Limits/2(phi_shin)
  PS-Simulink Converter/1 -> Angle Range Map/1("[-pi, pi]")
  Shin Motor [Nm]/1 -> Shin SEA/1(Shin Gear Torque [Nm])
  "Thigh Motor [Nm]  "/1 -> Thigh SEA/1(Thigh Gear Torque [Nm])
  connections:
  Simulink-PS Converter1/RConn1 -- External Force and Torque2/LConn1
  PS-Simulink Converter2/LConn1 -- Thigh Joint/RConn2
  PS-Simulink Converter3/LConn1 -- Thigh Joint/RConn3
  Flip Rotation Direction/RConn1 -- Rotate Frame 180 degrees/LConn1
  Thigh/LConn1 -- Flip Rotation Direction 2/RConn1
  Shin/LConn1 -- Flip Rotation Direction 1/RConn1
  Flip Rotation Direction/LConn1 -- Hip Conn/RConn1
  Thigh Joint/LConn1 -- Thigh SEA/LConn1 -- Shin Joint/LConn1 -- Shin SEA/LConn1 -- Rotate Frame 180 degrees/RConn1
  PS-Simulink Converter1/LConn1 -- Shin Joint/RConn3
  PS-Simulink Converter/LConn1 -- Shin Joint/RConn2
  Simulink-PS Converter/RConn1 -- External Force and Torque1/LConn1
  Shin/RConn1 -- Posterior Knee/LConn1
  External Force and Torque2/RConn1 -- Flip Rotation Direction 2/LConn1 -- Thigh Joint/RConn1
  External Force and Torque1/RConn1 -- Flip Rotation Direction 1/LConn1 -- Shin Joint/RConn1
  Thigh/RConn1 -- Anterior Knee/LConn1
  Lower Leg/LConn1 -- Anterior Knee/RConn1
  Lower Leg/RConn2 -- Foot Point/RConn1
  Four Bar Link/RConn1 -- Four Bar Link Joint/RConn1
  Four Bar Link/LConn1 -- Posterior Knee/RConn1
  Lower Leg/RConn1 -- Four Bar Link Joint/LConn1

== system atrias_boom_nmSt_kinSw_v2/Mechanical System Layer/Right Foot ==
  Ankle : sm_lib/Joints/Revolute Joint  SenseConstraintForce=off  SenseConstraintForceX=off  SenseConstraintForceY=off  SenseConstraintForceZ=off  SenseConstraintTorque=off  SenseConstraintTorqueX=off  SenseConstraintTorqueY=off  SenseConstraintTorqueZ=off  SenseTotalForce=off  SenseTotalForceX=off  SenseTotalForceY=off  SenseTotalForceZ=off  SenseTotalTorque=off  SenseTotalTorqueX=off  SenseTotalTorqueY=off  SenseTotalTorqueZ=off  CompositeWrenchDir=FollowerOnBase  CompositeWrenchFrame=BaseFrame  EquilibriumPosition=ankle_equilibrium  EquilibriumPositionUnits=rad  SpringStiffness=ankle_stiffness  SpringStiffnessUnits=N*m/rad  DampingCoefficient=0.1*ankle_stiffness  DampingCoefficientUnits=N*m/(rad/s)  TorqueActuationMode=NoTorque  MotionActuationMode=ComputedMotion  SensePosition=off  SenseVelocity=off  SenseAcceleration=off  SenseTorqueForce=off  PositionTargetSpecify=on  PositionTargetPriority=Low  PositionTargetValue=ankle_initial_r  PositionTargetValueUnits=rad  VelocityTargetSpecify=off  VelocityTargetPriority=High  VelocityTargetValue=6000  VelocityTargetValueUnits=deg/s  BlockFunction=simmechanics.library.joints.revolute_joint
  CS1 to Back Point : sm_lib/Frames and Transforms/Rigid Transform  TranslationMethod=Cartesian  TranslationLengthUnit=m  TranslationStandardAxis=+Z  TranslationStandardOffset=0  TranslationCartesianOffset=d_foot_point_back  TranslationROffset=0  TranslationROffsetUnits=m  TranslationZOffset=0  TranslationZOffsetUnits=m  TranslationThetaOffset=0  TranslationThetaOffsetUnits=deg  RotationMethod=None  RotationAngleUnits=deg  RotationStandardAxis=+Z  RotationAngle=0  RotationArbitraryAxis=[0 0 1]  FollAlignAxisA=+X  BaseAlignAxisA=+Y  FollAlignAxisB=+Y  BaseAlignAxisB=+Z  RotationMatrix=[1 0 0; 0 1 0; 0 0 1]  BlockFunction=simmechanics.library.frames_transforms.rigid_transform
  CS1 to Front Point : sm_lib/Frames and Transforms/Rigid Transform  TranslationMethod=Cartesian  TranslationLengthUnit=m  TranslationStandardAxis=+Z  TranslationStandardOffset=0  TranslationCartesianOffset=d_foot_point_front  TranslationROffset=0  TranslationROffsetUnits=m  TranslationZOffset=0  TranslationZOffsetUnits=m  TranslationThetaOffset=0  TranslationThetaOffsetUnits=deg  RotationMethod=None  RotationAngleUnits=deg  RotationStandardAxis=+Z  RotationAngle=0  RotationArbitraryAxis=[0 0 1]  FollAlignAxisA=+X  BaseAlignAxisA=+Y  FollAlignAxisB=+Y  BaseAlignAxisB=+Z  RotationMatrix=[1 0 0; 0 1 0; 0 0 1]  BlockFunction=simmechanics.library.frames_transforms.rigid_transform
  Solid : sm_lib/Body Elements/Solid  InertiaType=Custom  Mass=m_foot  MassUnits=kg  CenterOfMass=com_foot  CenterOfMassUnits=m  MomentsOfInertia=i_foot_moments  MomentsOfInertiaUnits=kg*m^2  ProductsOfInertia=i_foot_products  ProductsOfInertiaUnits=kg*m^2  DensityBased=on  Density=1000  DensityUnits=kg/(m^3)  GraphicType=FromGeometry  MarkerShape=Sphere  MarkerSize=10  MarkerSizeUnits=m  GraphicVisPropType=AdvancedVisualProperties  GraphicDiffuseColor=foot_color_d  GraphicSpecularColor=[0.5 0.5 0.5 1.0]  GraphicAmbientColor=[foot_color_d*0.5 1.0]  GraphicEmissiveColor=[0.0 0.0 0.0 1.0]  GraphicShininess=128  GraphicOpacity=1.0  GeometryShape=FromFile  RectangleSize=[1 1]  RectangleSizeUnits=m  BrickDimensions=[0.1 l_seg 0.1]  BrickDimensionUnits=m  CylinderRadius=l_rad  CylinderRadiusUnits=m  CylinderLength=l_seg  CylinderLengthUnits=m  SphereRadius=1  SphereRadiusUnits=m  EllipsoidRadii=[1 1 1]  EllipsoidRadiiUnits=m  ExtrusionCrossSection=[1 1; -1 1; -1 -1; 1 -1]  ExtrusionCrossSectionUnits=m  ExtrusionLength=1  ExtrusionLengthUnits=m  PolygonNumSides=3  PolygonOuterRadius=1  PolygonOuterRadiusUnits=m  ExtGeomFileType=STL  ExtGeomFileName=../models/foot.stl  ExtGeomFileUnits=m  RevolutionCrossSection=[1 1; 1 -1; 2 -1; 2 1]  RevolutionCrossSectionUnits=m  RevolutionExtent=Full  RevolutionAngle=180  RevolutionAngleUnits=deg  BlockFunction=simmechanics.library.body_elements.solid
  CS1 : PMIOPort  Port=1  Side=Left
  Back Point : PMIOPort  Port=2  Side=Right
  Front Point : PMIOPort  Port=3  Side=Right
  connections:
  Back Point/RConn1 -- CS1 to Back Point/RConn1
  CS1 to Back Point/LConn1 -- Ankle/RConn1 -- Solid/RConn1 -- CS1 to Front Point/LConn1
  Ankle/LConn1 -- CS1/RConn1
  Front Point/RConn1 -- CS1 to Front Point/RConn1
